simulink model "ADRCControl_CDPR_6DOF_20220708"  (R2020a)
settings: Solver=VariableStepAuto  StartTime=0.0  StopTime=12  RelTol=1e-3  EnableMultiTasking=on
values from neighbouring files (symbols this model uses):
  a = 25    [parameters_initialization.m]
  b = 0.05    [parameters_initialization.m]
  Kd = 7.062    [parameters_initialization.m]
  Kp = 70    [parameters_initialization.m]
undefined symbols (not defined in the file or in its folder): X, Y, Z
libraries: sm_lib x150, nesl_utility x52, sm_cable_robot_lib x30, simulink x1
(part 1 of 8)
settings Model: Creator=彭学东  LastModifiedBy=Administrator
settings DataIOCC: LimitDataPoints=on  MaxDataPoints=10000
settings OptimizationCC: LifeSpan=inf
settings DebuggingCC: AllowSymbolicDim=off  SFUnexpectedBacktrackingDiag=warning  SFNoUnconditionalDefaultTransitionDiag=warning  SFExecutionAtInitializationDiag=none  ArithmeticOperatorsInVariantConditions=warning
settings SFSimCC: SimUseLocalCustomCode=off  CustomCodeUndefinedFunction=UseInterfaceOnly
settings RTWCC: RTWUseLocalCustomCode=off
settings CodeAppCC: StateflowObjectComments=on
settings GRTTargetCC: TargetLangStandard=C89/C90 (ANSI)
settings ConfigComp: CovMetricSettings=dw  CovSaveCumulativeToWorkspaceVar=on  CovSaveSingleToWorkspaceVar=on  CovExternalEMLEnable=off  CovSFcnEnable=off
settings SimscapeCC: SimscapeLogType=all  SimscapeLogSimulationStatistics=on  SimscapeLogDataHistory=10000

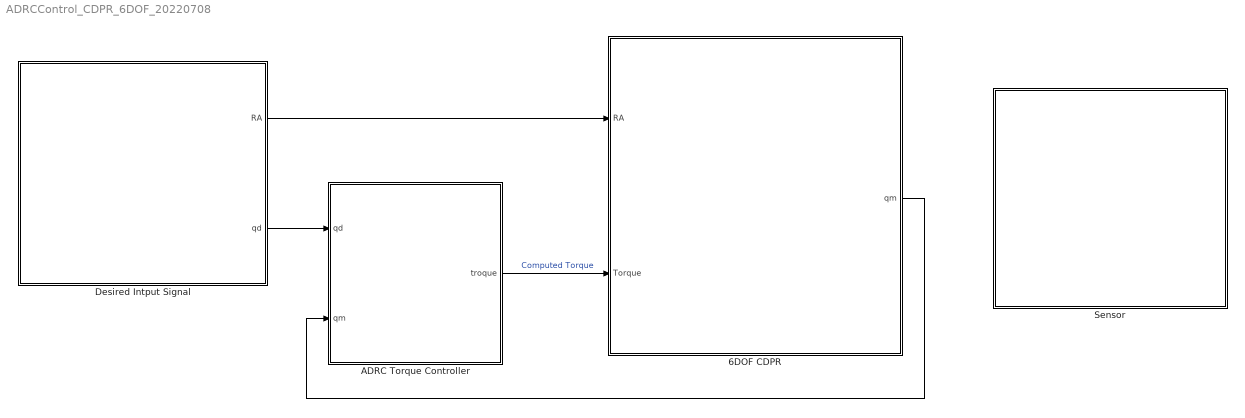
== system ADRCControl_CDPR_6DOF_20220708 ==
  6DOF CDPR : Subsystem
  ADRC Torque Controller : Subsystem
  Desired Intput Signal : Subsystem
  Sensor : Subsystem
  wires:
  Desired Intput Signal/2(qd) -> ADRC Torque Controller/1(qd)
  6DOF CDPR/1(qm) -> ADRC Torque Controller/2(qm)
  ADRC Torque Controller/1(troque) -> 6DOF CDPR/2(Torque)  "Computed Torque"
  Desired Intput Signal/1(RA) -> 6DOF CDPR/1(RA)

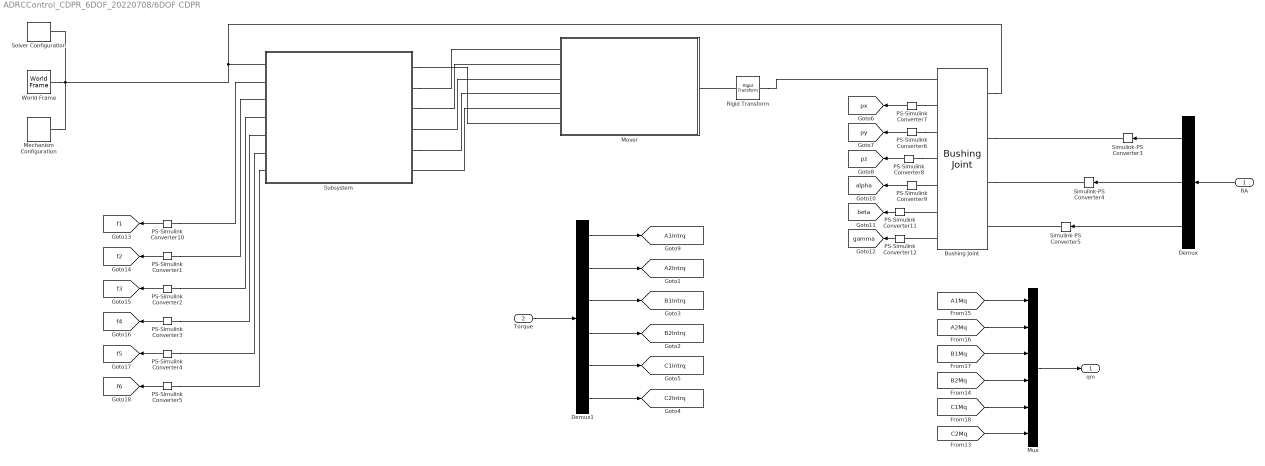
== system ADRCControl_CDPR_6DOF_20220708/6DOF CDPR ==
  RA : Inport
  Torque : Inport  Port=2
  Bushing Joint : sm_lib/Joints/Bushing Joint  JointMode=Normal  SenseConstraintForce=off  SenseConstraintForceX=off  SenseConstraintForceY=off  SenseConstraintForceZ=off  SenseConstraintTorque=off  SenseConstraintTorqueX=off  SenseConstraintTorqueY=off  SenseConstraintTorqueZ=off  SenseTotalForce=off  SenseTotalForceX=off  SenseTotalForceY=off  SenseTotalForceZ=off  SenseTotalTorque=off  SenseTotalTorqueX=off  SenseTotalTorqueY=off  SenseTotalTorqueZ=off  CompositeWrenchDir=FollowerOnBase  CompositeWrenchFrame=BaseFrame  PxEquilibriumPosition=0  PxEquilibriumPositionUnits=m  PxSpringStiffness=0  PxSpringStiffnessUnits=N/m  PxDampingCoefficient=0.1  PxDampingCoefficientUnits=N/(m/s)  PxTorqueActuationMode=NoTorque  PxMotionActuationMode=ComputedMotion  PxSensePosition=on  PxSenseVelocity=off  PxSenseAcceleration=off  PxSenseTorqueForce=off  PxSenseLowerLimitTorqueForce=off  PxSenseUpperLimitTorqueForce=off  PxLowerLimitSpecify=off  PxLowerLimitBound=-1  PxLowerLimitBoundUnits=m  PxLowerLimitStiffness=1e6  PxLowerLimitStiffnessUnits=N/m  PxLowerLimitDamping=1e3  PxLowerLimitDampingUnits=N/(m/s)  PxLowerLimitTransitionRegionWidth=1e-4  PxLowerLimitTransitionRegionWidthUnits=m  PxUpperLimitSpecify=off  PxUpperLimitBound=1  PxUpperLimitBoundUnits=m  PxUpperLimitStiffness=1e6  PxUpperLimitStiffnessUnits=N/m  PxUpperLimitDamping=1e3  PxUpperLimitDampingUnits=N/(m/s)  PxUpperLimitTransitionRegionWidth=1e-4  PxUpperLimitTransitionRegionWidthUnits=m  PxPositionTargetSpecify=on  PxPositionTargetPriority=High  PxPositionTargetValue=0.2  PxPositionTargetValueUnits=m  PxVelocityTargetSpecify=off  PxVelocityTargetPriority=High  PxVelocityTargetValue=0  PxVelocityTargetValueUnits=m/s  PyEquilibriumPosition=0  PyEquilibriumPositionUnits=m  PySpringStiffness=0  PySpringStiffnessUnits=N/m  PyDampingCoefficient=0.1  PyDampingCoefficientUnits=N/(m/s)  PyTorqueActuationMode=NoTorque  PyMotionActuationMode=ComputedMotion  PySensePosition=on  PySenseVelocity=off  PySenseAcceleration=off  PySenseTorqueForce=off  PySenseLowerLimitTorqueForce=off  PySenseUpperLimitTorqueForce=off  PyLowerLimitSpecify=off  PyLowerLimitBound=-1  PyLowerLimitBoundUnits=m  PyLowerLimitStiffness=1e6  PyLowerLimitStiffnessUnits=N/m  PyLowerLimitDamping=1e3  PyLowerLimitDampingUnits=N/(m/s)  PyLowerLimitTransitionRegionWidth=1e-4  PyLowerLimitTransitionRegionWidthUnits=m  PyUpperLimitSpecify=off  PyUpperLimitBound=1  PyUpperLimitBoundUnits=m  PyUpperLimitStiffness=1e6  PyUpperLimitStiffnessUnits=N/m  PyUpperLimitDamping=1e3  PyUpperLimitDampingUnits=N/(m/s)  PyUpperLimitTransitionRegionWidth=1e-4  PyUpperLimitTransitionRegionWidthUnits=m  PyPositionTargetSpecify=on  PyPositionTargetPriority=High  PyPositionTargetValue=0  PyPositionTargetValueUnits=m  PyVelocityTargetSpecify=off  PyVelocityTargetPriority=High  PyVelocityTargetValue=0  PyVelocityTargetValueUnits=m/s  PzEquilibriumPosition=0  PzEquilibriumPositionUnits=m  PzSpringStiffness=0  PzSpringStiffnessUnits=N/m  PzDampingCoefficient=0.1  PzDampingCoefficientUnits=N/(m/s)  PzTorqueActuationMode=NoTorque  PzMotionActuationMode=ComputedMotion  PzSensePosition=on  PzSenseVelocity=off  PzSenseAcceleration=off  PzSenseTorqueForce=off  PzSenseLowerLimitTorqueForce=off  PzSenseUpperLimitTorqueForce=off  PzLowerLimitSpecify=off  PzLowerLimitBound=-1  PzLowerLimitBoundUnits=m  PzLowerLimitStiffness=1e6  PzLowerLimitStiffnessUnits=N/m  PzLowerLimitDamping=1e3  PzLowerLimitDampingUnits=N/(m/s)  PzLowerLimitTransitionRegionWidth=1e-4  PzLowerLimitTransitionRegionWidthUnits=m  PzUpperLimitSpecify=off  PzUpperLimitBound=1  PzUpperLimitBoundUnits=m  PzUpperLimitStiffness=1e6  PzUpperLimitStiffnessUnits=N/m  PzUpperLimitDamping=1e3  PzUpperLimitDampingUnits=N/(m/s)  PzUpperLimitTransitionRegionWidth=1e-4  PzUpperLimitTransitionRegionWidthUnits=m  PzPositionTargetSpecify=on  PzPositionTargetPriority=High  PzPositionTargetValue=1.3  PzPositionTargetValueUnits=m  PzVelocityTargetSpecify=off  PzVelocityTargetPriority=High  PzVelocityTargetValue=0  PzVelocityTargetValueUnits=m/s  RxEquilibriumPosition=0  RxEquilibriumPositionUnits=deg  RxSpringStiffness=0  RxSpringStiffnessUnits=N*m/deg  RxDampingCoefficient=0.1  RxDampingCoefficientUnits=N*m/(deg/s)  RxTorqueActuationMode=ComputedTorque  RxMotionActuationMode=InputMotion  RxSensePosition=on  RxSenseVelocity=off  RxSenseAcceleration=off  RxSenseTorqueForce=off  RxSenseLowerLimitTorqueForce=off  RxSenseUpperLimitTorqueForce=off  RxLowerLimitSpecify=off  RxLowerLimitBound=-90  RxLowerLimitBoundUnits=deg  RxLowerLimitStiffness=1e4  RxLowerLimitStiffnessUnits=N*m/deg  RxLowerLimitDamping=10  RxLowerLimitDampingUnits=N*m/(deg/s)  RxLowerLimitTransitionRegionWidth=0.1  RxLowerLimitTransitionRegionWidthUnits=deg  RxUpperLimitSpecify=off  RxUpperLimitBound=90  RxUpperLimitBoundUnits=deg  RxUpperLimitStiffness=1e4  RxUpperLimitStiffnessUnits=N*m/deg  RxUpperLimitDamping=10  RxUpperLimitDampingUnits=N*m/(deg/s)  RxUpperLimitTransitionRegionWidth=0.1  RxUpperLimitTransitionRegionWidthUnits=deg  RxPositionTargetSpecify=off  RxPositionTargetPriority=High  RxPositionTargetValue=0  RxPositionTargetValueUnits=deg  RxVelocityTargetSpecify=off  RxVelocityTargetPriority=High  RxVelocityTargetValue=0  RxVelocityTargetValueUnits=deg/s  RyEquilibriumPosition=0  RyEquilibriumPositionUnits=deg  RySpringStiffness=0  RySpringStiffnessUnits=N*m/deg  RyDampingCoefficient=0.1  RyDampingCoefficientUnits=N*m/(deg/s)  RyTorqueActuationMode=ComputedTorque  RyMotionActuationMode=InputMotion  RySensePosition=on  RySenseVelocity=off  RySenseAcceleration=off  RySenseTorqueForce=off  RySenseLowerLimitTorqueForce=off  RySenseUpperLimitTorqueForce=off  RyLowerLimitSpecify=off  RyLowerLimitBound=-90  RyLowerLimitBoundUnits=deg  RyLowerLimitStiffness=1e4  RyLowerLimitStiffnessUnits=N*m/deg  RyLowerLimitDamping=10  RyLowerLimitDampingUnits=N*m/(deg/s)  RyLowerLimitTransitionRegionWidth=0.1  RyLowerLimitTransitionRegionWidthUnits=deg  RyUpperLimitSpecify=off  RyUpperLimitBound=90  RyUpperLimitBoundUnits=deg  RyUpperLimitStiffness=1e4  RyUpperLimitStiffnessUnits=N*m/deg  RyUpperLimitDamping=10  RyUpperLimitDampingUnits=N*m/(deg/s)  RyUpperLimitTransitionRegionWidth=0.1  RyUpperLimitTransitionRegionWidthUnits=deg  RyPositionTargetSpecify=off  RyPositionTargetPriority=High  RyPositionTargetValue=0  RyPositionTargetValueUnits=deg  RyVelocityTargetSpecify=off  RyVelocityTargetPriority=High  RyVelocityTargetValue=0  RyVelocityTargetValueUnits=deg/s  RzEquilibriumPosition=0  RzEquilibriumPositionUnits=deg  RzSpringStiffness=0  RzSpringStiffnessUnits=N*m/deg  RzDampingCoefficient=0.1  RzDampingCoefficientUnits=N*m/(deg/s)  RzTorqueActuationMode=ComputedTorque  RzMotionActuationMode=InputMotion  RzSensePosition=on  RzSenseVelocity=off  RzSenseAcceleration=off  RzSenseTorqueForce=off  RzSenseLowerLimitTorqueForce=off  RzSenseUpperLimitTorqueForce=off  RzLowerLimitSpecify=off  RzLowerLimitBound=-90  RzLowerLimitBoundUnits=deg  RzLowerLimitStiffness=1e4  RzLowerLimitStiffnessUnits=N*m/deg  RzLowerLimitDamping=10  RzLowerLimitDampingUnits=N*m/(deg/s)  RzLowerLimitTransitionRegionWidth=0.1  RzLowerLimitTransitionRegionWidthUnits=deg  RzUpperLimitSpecify=off  RzUpperLimitBound=90  RzUpperLimitBoundUnits=deg  RzUpperLimitStiffness=1e4  RzUpperLimitStiffnessUnits=N*m/deg  RzUpperLimitDamping=10  RzUpperLimitDampingUnits=N*m/(deg/s)  RzUpperLimitTransitionRegionWidth=0.1  RzUpperLimitTransitionRegionWidthUnits=deg  RzPositionTargetSpecify=off  RzPositionTargetPriority=High  RzPositionTargetValue=0  RzPositionTargetValueUnits=deg  RzVelocityTargetSpecify=off  RzVelocityTargetPriority=High  RzVelocityTargetValue=0  RzVelocityTargetValueUnits=deg/s
  Demux : Demux  Outputs=3
  Demux1 : Demux  Outputs=6
  Mechanism Configuration : sm_lib/Utilities/Mechanism Configuration  UniformGravity=Constant  GravityVector=[0 0 -9.80665]  GravityUnits=m/s^2  LinearizationDelta=0.001
  Mover : Subsystem
  Mux : Mux  Inputs=6
  PS-Simulink Converter{1..12} (12 alike) : nesl_utility/PS-Simulink Converter  PhysicalDomain=network_engine_domain  SubClassName=ps_output  LeftPortType=input  RightPortType=output  PseudoPeriodic=off  Frequencies=[]  Unit=inherit  AffineConversion=off
  Rigid Transform : sm_lib/Frames and Transforms/Rigid Transform  TranslationMethod=None  TranslationStandardOffset=0  TranslationLengthUnit=m  TranslationStandardAxis=+Z  TranslationCartesianOffset=[0 0 0]  TranslationROffset=0  TranslationROffsetUnits=m  TranslationZOffset=0  TranslationZOffsetUnits=m  TranslationThetaOffset=0  TranslationThetaOffsetUnits=deg  RotationMethod=ArbitraryAxis  RotationAngleUnits=deg  RotationStandardAxis=+Z  RotationAngle=120.0  RotationArbitraryAxis=[0 0 1]  FollAlignAxisA=+X  BaseAlignAxisA=+Y  FollAlignAxisB=+Y  BaseAlignAxisB=+Z  RotationSequenceAxes=FollowerAxes  RotationSequence=XYX  RotationSequenceAngles=[0 0 0]  RotationSequenceAnglesUnits=deg  RotationMatrix=[1 0 0; 0 1 0; 0 0 1]
  Simulink-PS Converter3 : nesl_utility/Simulink-PS Converter  PhysicalDomain=network_engine_domain  SubClassName=ps_input  LeftPortType=input  RightPortType=output  PseudoPeriodic=off  Frequencies=[]  NoiseDistribution=none  NoiseParameters=[]  Unit=1  AffineConversion=off  FilteringAndDerivatives=filter  SimscapeFilterOrder=2  InputFilterTimeConstant=0.001  UdotUserProvided=0
  Simulink-PS Converter4 : nesl_utility/Simulink-PS Converter  PhysicalDomain=network_engine_domain  SubClassName=ps_input  LeftPortType=input  RightPortType=output  PseudoPeriodic=off  Frequencies=[]  NoiseDistribution=none  NoiseParameters=[]  Unit=1  AffineConversion=off  FilteringAndDerivatives=filter  SimscapeFilterOrder=2  InputFilterTimeConstant=0.001  UdotUserProvided=0
  Simulink-PS Converter5 : nesl_utility/Simulink-PS Converter  PhysicalDomain=network_engine_domain  SubClassName=ps_input  LeftPortType=input  RightPortType=output  PseudoPeriodic=off  Frequencies=[]  NoiseDistribution=none  NoiseParameters=[]  Unit=1  AffineConversion=off  FilteringAndDerivatives=filter  SimscapeFilterOrder=2  InputFilterTimeConstant=0.001  UdotUserProvided=0
  Solver Configuration : nesl_utility/Solver Configuration  PhysicalDomain=network_engine_domain  SubClassName=solver  LeftPortType=input  RightPortType=generic  Tones=[]  Harmonics=[]  SimulateNoise=off  Profile=off  UseLocalSampling=off  EnableSwitchedLinearOptims=on  FrequencyDomain=off  UseCCode=off  RelTol=0.001  AbsTol=1e-06  MinStep=1e-09  ToWorkspace=off  RevertToSquareIcSolve=off  NumHomotopyIterations=100  PhasorMode=off  PhasorModeNumHarmonics=1  DoDC=off  ResidualTolerance=1e-01  UseLocalSolver=off  LocalSolverChoice=NE_BACKWARD_EULER_ADVANCER  LocalSolverSampleTime=0.001  DoFixedCost=off  MaxNonlinIter=3  MaxModeIter=2  LinearAlgebra=Sparse  EquationFormulation=NE_TIME_EF  DelaysMemoryBudget=1024  AutomaticFiltering=on  FilteringTimeConstant=0.001  PartitionStorageMethod=AS_NEEDED  PartitionMemoryBudget=1024  PartitionMethod=FAST
  Subsystem : Subsystem
  World Frame : sm_lib/Frames and Transforms/World Frame
  qm : Outport
  tag scope: A1Intrq=global, A2Intrq=global, B1Intrq=global, B2Intrq=global, C1Intrq=global, C2Intrq=global, alpha=global, beta=global, f1=global, f2=global, f3=global, f4=global, f5=global, f6=global, gamma=global, px=global, py=global, pz=global
  wires:
  PS-Simulink Converter9/1 -> [alpha]
  PS-Simulink Converter3/1 -> [f4]
  Demux1/1 -> [A1Intrq]
  Demux1/5 -> [C1Intrq]
  PS-Simulink Converter7/1 -> [px]
  PS-Simulink Converter1/1 -> [f2]
  Torque/1 -> Demux1/1
  Demux/2 -> Simulink-PS Converter4/1
  Demux/1 -> Simulink-PS Converter3/1
  PS-Simulink Converter10/1 -> [f1]
  Demux/3 -> Simulink-PS Converter5/1
  Demux1/3 -> [B1Intrq]
  PS-Simulink Converter11/1 -> [beta]
  PS-Simulink Converter8/1 -> [pz]
  Demux1/6 -> [C2Intrq]
  Demux1/2 -> [A2Intrq]
  PS-Simulink Converter2/1 -> [f3]
  PS-Simulink Converter12/1 -> [gamma]
  PS-Simulink Converter4/1 -> [f5]
  RA/1 -> Demux/1
  PS-Simulink Converter5/1 -> [f6]
  PS-Simulink Converter6/1 -> [py]
  Demux1/4 -> [B2Intrq]
  [B1Mq] -> Mux/3
  [A2Mq] -> Mux/2
  [C1Mq] -> Mux/5
  [A1Mq] -> Mux/1
  [C2Mq] -> Mux/6
  [B2Mq] -> Mux/4
  Mux/1 -> qm/1
  connections:
  World Frame/RConn1 -- Bushing Joint/LConn1 -- Subsystem/LConn1 -- Mechanism Configuration/RConn1 -- Solver Configuration/RConn1
  Subsystem/RConn2 -- Mover/LConn1
  Mover/LConn5 -- Subsystem/RConn6
  Bushing Joint/RConn6 -- PS-Simulink Converter11/LConn1
  Bushing Joint/RConn7 -- PS-Simulink Converter12/LConn1
  Rigid Transform/LConn1 -- Mover/RConn1
  PS-Simulink Converter10/LConn1 -- Subsystem/LConn2
  Bushing Joint/LConn2 -- Simulink-PS Converter3/RConn1
  Mover/LConn3 -- Subsystem/RConn4
  Subsystem/RConn5 -- Mover/LConn4
  Subsystem/RConn3 -- Mover/LConn2
  PS-Simulink Converter2/LConn1 -- Subsystem/LConn4
  PS-Simulink Converter4/LConn1 -- Subsystem/LConn6
  PS-Simulink Converter8/LConn1 -- Bushing Joint/RConn4
  PS-Simulink Converter5/LConn1 -- Subsystem/LConn7
  Bushing Joint/RConn5 -- PS-Simulink Converter9/LConn1
  PS-Simulink Converter1/LConn1 -- Subsystem/LConn3
  PS-Simulink Converter3/LConn1 -- Subsystem/LConn5
  Rigid Transform/RConn1 -- Bushing Joint/RConn1
  Subsystem/RConn1 -- Mover/LConn6
  PS-Simulink Converter7/LConn1 -- Bushing Joint/RConn2
  Bushing Joint/LConn3 -- Simulink-PS Converter4/RConn1
  PS-Simulink Converter6/LConn1 -- Bushing Joint/RConn3
  Simulink-PS Converter5/RConn1 -- Bushing Joint/LConn4

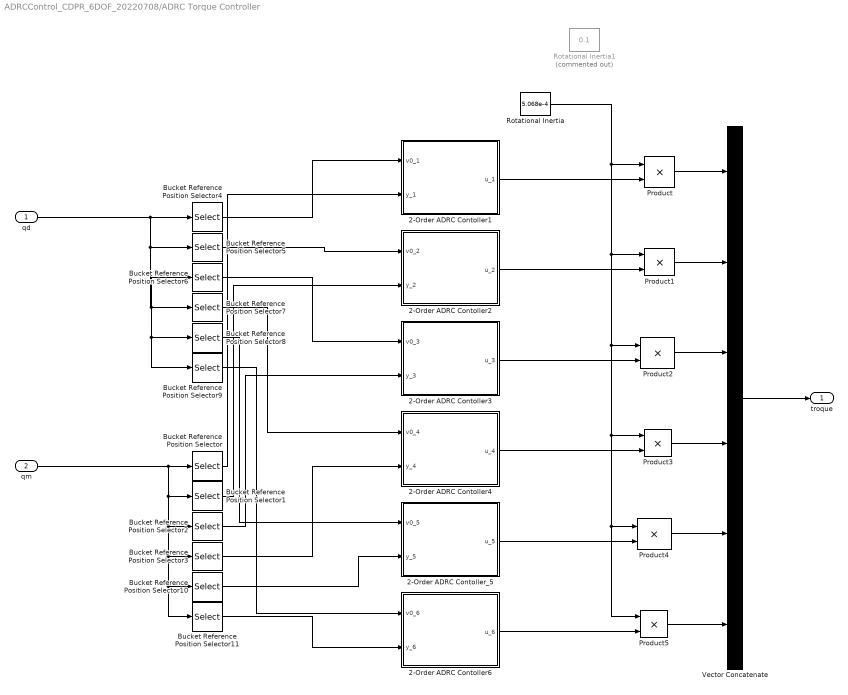
== system ADRCControl_CDPR_6DOF_20220708/ADRC Torque Controller ==
  qd : Inport
  qm : Inport  Port=2
  "2-Order ADRC Contoller1 " : Subsystem
  2-Order ADRC Contoller2 : Subsystem
  2-Order ADRC Contoller3 : Subsystem
  2-Order ADRC Contoller4 : Subsystem
  2-Order ADRC Contoller6 : Subsystem
  2-Order ADRC Contoller_5 : Subsystem
  Bucket Reference Position Selector : Selector  InputPortWidth=6  IndexOptions=Index vector (dialog)  Indices=1  OutputSizes=1
  Bucket Reference Position Selector1 : Selector  InputPortWidth=6  IndexOptions=Index vector (dialog)  Indices=2  OutputSizes=1
  Bucket Reference Position Selector10 : Selector  InputPortWidth=6  IndexOptions=Index vector (dialog)  Indices=5  OutputSizes=1
  Bucket Reference Position Selector11 : Selector  InputPortWidth=6  IndexOptions=Index vector (dialog)  Indices=6  OutputSizes=1
  Bucket Reference Position Selector2 : Selector  InputPortWidth=6  IndexOptions=Index vector (dialog)  Indices=3  OutputSizes=1
  Bucket Reference Position Selector3 : Selector  InputPortWidth=6  IndexOptions=Index vector (dialog)  Indices=4  OutputSizes=1
  Bucket Reference Position Selector4 : Selector  InputPortWidth=6  IndexOptions=Index vector (dialog)  Indices=1  OutputSizes=1
  Bucket Reference Position Selector5 : Selector  InputPortWidth=6  IndexOptions=Index vector (dialog)  Indices=2  OutputSizes=1
  Bucket Reference Position Selector6 : Selector  InputPortWidth=6  IndexOptions=Index vector (dialog)  Indices=3  OutputSizes=1
  Bucket Reference Position Selector7 : Selector  InputPortWidth=6  IndexOptions=Index vector (dialog)  Indices=4  OutputSizes=1
  Bucket Reference Position Selector8 : Selector  InputPortWidth=6  IndexOptions=Index vector (dialog)  Indices=5  OutputSizes=1
  Bucket Reference Position Selector9 : Selector  InputPortWidth=6  IndexOptions=Index vector (dialog)  Indices=6  OutputSizes=1
  Product{,1..5} (6 alike) : Product
  Rotational Inertia : Constant  Value=5.068e-4
  Rotational Inertia1 : Constant  Commented=on  Value=0.1
  Vector Concatenate : Concatenate  NumInputs=6
  troque : Outport  VectorParamsAs1DForOutWhenUnconnected=off
  wires:
  Vector Concatenate/1 -> troque/1
  Rotational Inertia/1 -> Product/1, Product1/1, Product2/1, Product3/1, Product5/1, Product4/1
  Product/1 -> Vector Concatenate/1
  Product1/1 -> Vector Concatenate/2
  Product2/1 -> Vector Concatenate/3
  Product3/1 -> Vector Concatenate/4
  "2-Order ADRC Contoller1 "/1(u_1) -> Product/2
  2-Order ADRC Contoller2/1(u_2) -> Product1/2
  2-Order ADRC Contoller3/1(u_3) -> Product2/2
  2-Order ADRC Contoller4/1(u_4) -> Product3/2
  qm/1 -> Bucket Reference Position Selector11/1, Bucket Reference Position Selector10/1, Bucket Reference Position Selector3/1, Bucket Reference Position Selector2/1, Bucket Reference Position Selector1/1, Bucket Reference Position Selector/1
  qd/1 -> Bucket Reference Position Selector9/1, Bucket Reference Position Selector8/1, Bucket Reference Position Selector7/1, Bucket Reference Position Selector6/1, Bucket Reference Position Selector5/1, Bucket Reference Position Selector4/1
  Bucket Reference Position Selector4/1 -> "2-Order ADRC Contoller1 "/1(v0_1)
  Bucket Reference Position Selector5/1 -> 2-Order ADRC Contoller2/1(v0_2)
  Bucket Reference Position Selector6/1 -> 2-Order ADRC Contoller3/1(v0_3)
  Bucket Reference Position Selector7/1 -> 2-Order ADRC Contoller4/1(v0_4)
  Bucket Reference Position Selector/1 -> "2-Order ADRC Contoller1 "/2(y_1)
  Bucket Reference Position Selector1/1 -> 2-Order ADRC Contoller2/2(y_2)
  Bucket Reference Position Selector2/1 -> 2-Order ADRC Contoller3/2(y_3)
  Bucket Reference Position Selector3/1 -> 2-Order ADRC Contoller4/2(y_4)
  Bucket Reference Position Selector8/1 -> 2-Order ADRC Contoller_5/1(v0_5)
  Bucket Reference Position Selector9/1 -> 2-Order ADRC Contoller6/1(v0_6)
  Bucket Reference Position Selector10/1 -> 2-Order ADRC Contoller_5/2(y_5)
  Bucket Reference Position Selector11/1 -> 2-Order ADRC Contoller6/2(y_6)
  Product5/1 -> Vector Concatenate/6
  2-Order ADRC Contoller_5/1(u_5) -> Product4/2
  2-Order ADRC Contoller6/1(u_6) -> Product5/2
  Product4/1 -> Vector Concatenate/5

== system ADRCControl_CDPR_6DOF_20220708/Desired Intput Signal ==
  Clock1 : Clock  Commented=on
      settings: Decimation=12
  Clock2 : Clock
      settings: Decimation=12
  Desried Angle : MATLAB Function  TreatAsAtomicUnit=on
  Desried Torque1 : MATLAB Function  Commented=on  TreatAsAtomicUnit=on
  Mux : Mux  Inputs=3
  Mux1 : Mux  Inputs=6
  Mux2 : Mux  Commented=on  Inputs=6
  Rotation Angle : Subsystem
  RA : Outport
  qd : Outport  Port=2
  wires:
  Rotation Angle/1(Out1) -> Mux/1
  Rotation Angle/2(Out2) -> Mux/2
  Rotation Angle/3(Out3) -> Mux/3
  Mux/1 -> RA/1
  Desried Angle/2(A2q) -> Mux1/2
  Desried Angle/6(C2q) -> Mux1/6
  Desried Angle/3(B1q) -> Mux1/3
  Clock2/1 -> Desried Angle/1(t)
  Desried Angle/1(A1q) -> Mux1/1
  Desried Angle/4(B2q) -> Mux1/4
  Desried Angle/5(C1q) -> Mux1/5
  Mux1/1 -> qd/1
  Desried Torque1/4(B2q) -> Mux2/4
  Desried Torque1/3(B1q) -> Mux2/3
  Desried Torque1/2(A2q) -> Mux2/2
  Desried Torque1/1(A1q) -> Mux2/1
  Desried Torque1/6(C2q) -> Mux2/6
  Desried Torque1/5(C1q) -> Mux2/5
  Clock1/1 -> Desried Torque1/1(t)

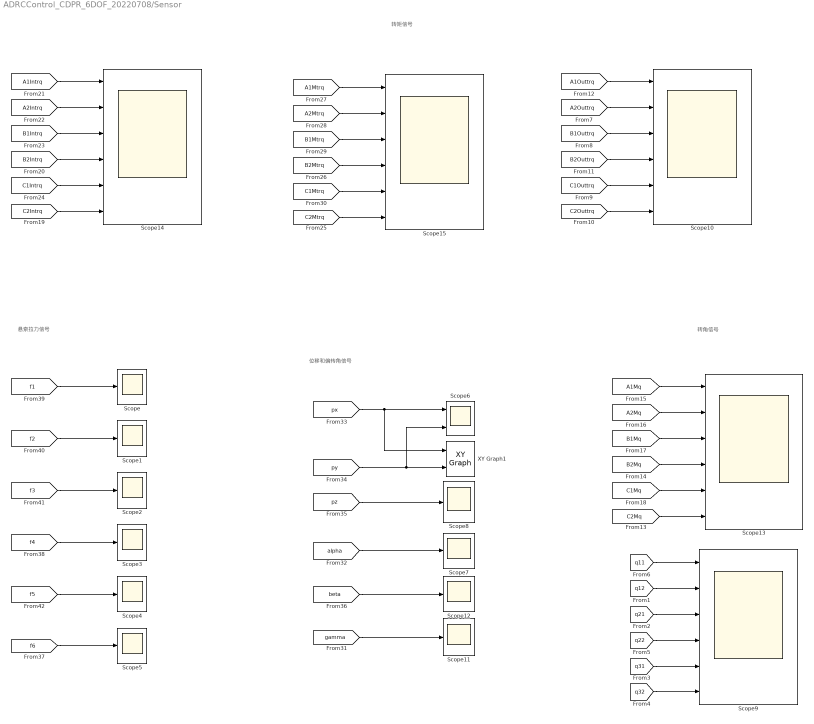
== system ADRCControl_CDPR_6DOF_20220708/Sensor ==
  note: 悬索拉力信号
  note: 位移和偏转角信号
  note: 转角信号
  note: 转矩信号
  Scope{,1..5,7..8,11..12} (10 alike) : Scope
  Scope{9..10,13..15} (5 alike) : Scope  NumInputPorts=6
  Scope6 : Scope  NumInputPorts=2
  XY Graph1 : simulink/Sinks/XY Graph  xmin=-1.1  xmax=1.1  ymin=-1.5  ymax=1.5  st=-1
  wires:
  [C2Outtrq] -> Scope10/6
  [C2Mtrq] -> Scope15/6
  [C1Intrq] -> Scope14/5
  [B2Intrq] -> Scope14/4
  [B1Mtrq] -> Scope15/3
  [C1Mtrq] -> Scope15/5
  [B1Intrq] -> Scope14/3
  [B2Mtrq] -> Scope15/4
  [A2Intrq] -> Scope14/2
  [A1Mtrq] -> Scope15/1
  [C1Outtrq] -> Scope10/5
  [A1Intrq] -> Scope14/1
  [C2Intrq] -> Scope14/6
  [B1Outtrq] -> Scope10/3
  [A2Outtrq] -> Scope10/2
  [A1Outtrq] -> Scope10/1
  [B2Outtrq] -> Scope10/4
  [A2Mtrq] -> Scope15/2
  [B1Mq] -> Scope13/3
  [B2Mq] -> Scope13/4
  [C2Mq] -> Scope13/6
  [q12] -> Scope9/2
  [q21] -> Scope9/3
  [C1Mq] -> Scope13/5
  [A1Mq] -> Scope13/1
  [q22] -> Scope9/4
  [q32] -> Scope9/6
  [q31] -> Scope9/5
  [q11] -> Scope9/1
  [A2Mq] -> Scope13/2
  [gamma] -> Scope11/1
  [beta] -> Scope12/1
  [alpha] -> Scope7/1
  [pz] -> Scope8/1
  [py] -> XY Graph1/2, Scope6/2
  [px] -> Scope6/1, XY Graph1/1
  [f1] -> Scope/1
  [f2] -> Scope1/1
  [f3] -> Scope2/1
  [f4] -> Scope3/1
  [f5] -> Scope4/1
  [f6] -> Scope5/1

== system ADRCControl_CDPR_6DOF_20220708/6DOF CDPR/Mover ==
  Extruded Solid : sm_lib/Body Elements/Extruded Solid  GraphicAmbientColor=[0.15 0.15 0.15 1.0]  BasedOnType=Mass  CenterOfMass=[0 0 0]  CenterOfMassUnits=m  GraphicDiffuseColor=[0.0 0.2 1.0]  ExportConvexHullGeometry=off  ExtrusionCrossSection=[1 1; -1 1; -1 -1; 1 -1]  ExtrusionCrossSectionUnits=m  Density=1000  DensityUnits=kg/m^3  DoExposeReferenceFrame=on  GraphicEmissiveColor=[0.0 0.0 0.0 1.0]  ExportEntireGeometry=off  ExtrusionLength=0.1  ExtrusionLengthUnits=m  ExtrusionType=Regular  SerializedFrames=<Frames><Frame><Id>Frame1</Id><Value><Name>F1</Name><Origin><Source>GeometricFeature</Source><FeatureName>side curve 3</FeatureName></Origin><PrimaryAxis><DefinedDirection>+Z</DefinedDirection><Source>ReferenceFrame</Source><SourceDirection>+Z</SourceDirection><FeatureName></FeatureName></PrimaryAxis><SecondaryAxis><DefinedDirection>+X</DefinedDirection><Source>ReferenceFrame</Source><SourceDirection>+X</SourceDirection><FeatureName></FeatureName></SecondaryAxis></Value></Frame><Frame><Id>Frame2</Id><Value><Name>F2</Name><Origin><Source>GeometricFeature</Source><FeatureName>side curve 1</FeatureName></Origin><PrimaryAxis><DefinedDirection>+Z</DefinedDirection><Source>ReferenceFrame</Source><SourceDirection>+Z</SourceDirection><FeatureName></FeatureName></PrimaryAxis><SecondaryAxis><DefinedDirection>+X</DefinedDirection><Source>ReferenceFrame</Source><SourceDirection>+X</SourceDirection><FeatureName></FeatureName></SecondaryAxis></Value></Frame><Frame><Id>Frame3</Id><Value><Name>F3</Name><Origin><Source>GeometricFeature</Source><FeatureName>side curve 2</FeatureName></Origin><PrimaryAxis><DefinedDirection>+Z</DefinedDirection><Source>ReferenceFrame</Source><SourceDirection>+Z</SourceDirection><FeatureName></FeatureName></PrimaryAxis><SecondaryAxis><DefinedDirection>+X</DefinedDirection><Source>ReferenceFrame</Source><SourceDirection>+X</SourceDirection><FeatureName></FeatureName></SecondaryAxis></Value></Frame></Frames>  MarkerShape=Sphere  MarkerSize=10  GraphicType=FromGeometry  InertiaType=Custom  Mass=5  MassUnits=kg  MomentsOfInertia=[0.001 0.001 0.03125]  MomentsOfInertiaUnits=kg*m^2  PolygonNumSides=3  GraphicOpacity=1.0  PolygonOuterRadius=0.088  PolygonOuterRadiusUnits=m  ProductsOfInertia=[0 0 0]  ProductsOfInertiaUnits=kg*m^2  GraphicShininess=75  GraphicSpecularColor=[0.5 0.5 0.5 1.0]  GraphicVisPropType=SimpleVisualProperties
  1 : PMIOPort  Side=Left
  2 : PMIOPort  Port=2  Side=Left
  3 : PMIOPort  Port=3  Side=Left
  4 : PMIOPort  Port=4  Side=Left
  5 : PMIOPort  Port=5  Side=Left
  6 : PMIOPort  Port=6  Side=Left
  B : PMIOPort  Port=7  Side=Right
  connections:
  5/RConn1 -- 6/RConn1 -- Extruded Solid/RConn2
  3/RConn1 -- 4/RConn1 -- Extruded Solid/LConn2
  2/RConn1 -- 1/RConn1 -- Extruded Solid/LConn1
  B/RConn1 -- Extruded Solid/RConn1

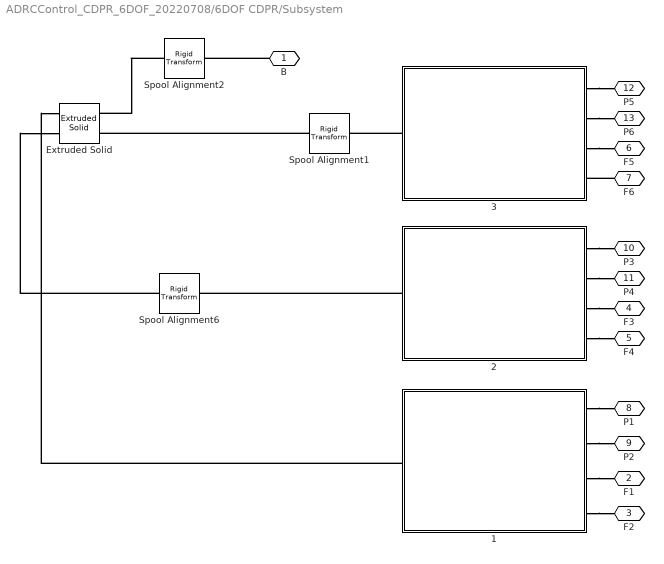
== system ADRCControl_CDPR_6DOF_20220708/6DOF CDPR/Subsystem ==
  1 : Subsystem
  2 : Subsystem
  3 : Subsystem
  Extruded Solid : sm_lib/Body Elements/Extruded Solid  GraphicAmbientColor=[0.15 0.15 0.15 1.0]  BasedOnType=Density  CenterOfMass=[0 0 0]  CenterOfMassUnits=m  GraphicDiffuseColor=[0.5 0.5 0.5]  ExportConvexHullGeometry=off  ExtrusionCrossSection=[1 1; -1 1; -1 -1; 1 -1]  ExtrusionCrossSectionUnits=m  Density=1000  DensityUnits=kg/m^3  DoExposeReferenceFrame=on  GraphicEmissiveColor=[0.0 0.0 0.0 1.0]  ExportEntireGeometry=off  ExtrusionLength=0.2  ExtrusionLengthUnits=m  ExtrusionType=Regular  SerializedFrames=<Frames><Frame><Id>Frame1</Id><Value><Name>F1</Name><Origin><Source>GeometricFeature</Source><FeatureName>top point 3</FeatureName></Origin><PrimaryAxis><DefinedDirection>+Z</DefinedDirection><Source>ReferenceFrame</Source><SourceDirection>+Z</SourceDirection><FeatureName></FeatureName></PrimaryAxis><SecondaryAxis><DefinedDirection>+X</DefinedDirection><Source>ReferenceFrame</Source><SourceDirection>+X</SourceDirection><FeatureName></FeatureName></SecondaryAxis></Value></Frame><Frame><Id>Frame2</Id><Value><Name>F2</Name><Origin><Source>GeometricFeature</Source><FeatureName>top point 1</FeatureName></Origin><PrimaryAxis><DefinedDirection>+Z</DefinedDirection><Source>ReferenceFrame</Source><SourceDirection>+Z</SourceDirection><FeatureName></FeatureName></PrimaryAxis><SecondaryAxis><DefinedDirection>+X</DefinedDirection><Source>ReferenceFrame</Source><SourceDirection>+X</SourceDirection><FeatureName></FeatureName></SecondaryAxis></Value></Frame><Frame><Id>Frame3</Id><Value><Name>F3</Name><Origin><Source>GeometricFeature</Source><FeatureName>top point 2</FeatureName></Origin><PrimaryAxis><DefinedDirection>+Z</DefinedDirection><Source>ReferenceFrame</Source><SourceDirection>+Z</SourceDirection><FeatureName></FeatureName></PrimaryAxis><SecondaryAxis><DefinedDirection>+X</DefinedDirection><Source>ReferenceFrame</Source><SourceDirection>+X</SourceDirection><FeatureName></FeatureName></SecondaryAxis></Value></Frame></Frames>  MarkerShape=Sphere  MarkerSize=10  GraphicType=FromGeometry  InertiaType=CalculateFromGeometry  Mass=1  MassUnits=kg  MomentsOfInertia=[1 1 1]  MomentsOfInertiaUnits=kg*m^2  PolygonNumSides=3  GraphicOpacity=1.0  PolygonOuterRadius=2.254  PolygonOuterRadiusUnits=m  ProductsOfInertia=[0 0 0]  ProductsOfInertiaUnits=kg*m^2  GraphicShininess=75  GraphicSpecularColor=[0.5 0.5 0.5 1.0]  GraphicVisPropType=SimpleVisualProperties
  Spool Alignment1 : sm_lib/Frames and Transforms/Rigid Transform  TranslationMethod=None  TranslationStandardOffset=0  TranslationLengthUnit=m  TranslationStandardAxis=+Z  TranslationCartesianOffset=[0 0 0]  TranslationROffset=0  TranslationROffsetUnits=m  TranslationZOffset=0  TranslationZOffsetUnits=m  TranslationThetaOffset=0  TranslationThetaOffsetUnits=deg  RotationMethod=ArbitraryAxis  RotationAngleUnits=deg  RotationStandardAxis=+Z  RotationAngle=-120.0  RotationArbitraryAxis=[0 0 1]  FollAlignAxisA=+X  BaseAlignAxisA=+X  FollAlignAxisB=+Y  BaseAlignAxisB=+Y  RotationSequenceAxes=FollowerAxes  RotationSequence=XYX  RotationSequenceAngles=[0 0 0]  RotationSequenceAnglesUnits=deg  RotationMatrix=[1 0 0; 0 1 0; 0 0 1]
  Spool Alignment2 : sm_lib/Frames and Transforms/Rigid Transform  TranslationMethod=None  TranslationStandardOffset=0  TranslationLengthUnit=m  TranslationStandardAxis=+Z  TranslationCartesianOffset=[0 0 0]  TranslationROffset=0  TranslationROffsetUnits=m  TranslationZOffset=0  TranslationZOffsetUnits=m  TranslationThetaOffset=0  TranslationThetaOffsetUnits=deg  RotationMethod=ArbitraryAxis  RotationAngleUnits=deg  RotationStandardAxis=+Z  RotationAngle=180.0  RotationArbitraryAxis=[0 0 1]  FollAlignAxisA=+X  BaseAlignAxisA=+X  FollAlignAxisB=+Y  BaseAlignAxisB=+Y  RotationSequenceAxes=FollowerAxes  RotationSequence=XYX  RotationSequenceAngles=[0 0 0]  RotationSequenceAnglesUnits=deg  RotationMatrix=[1 0 0; 0 1 0; 0 0 1]
  Spool Alignment6 : sm_lib/Frames and Transforms/Rigid Transform  TranslationMethod=None  TranslationStandardOffset=0  TranslationLengthUnit=m  TranslationStandardAxis=+Z  TranslationCartesianOffset=[0 0 0]  TranslationROffset=0  TranslationROffsetUnits=m  TranslationZOffset=0  TranslationZOffsetUnits=m  TranslationThetaOffset=0  TranslationThetaOffsetUnits=deg  RotationMethod=ArbitraryAxis  RotationAngleUnits=deg  RotationStandardAxis=+Z  RotationAngle=120.0  RotationArbitraryAxis=[0 0 1]  FollAlignAxisA=+X  BaseAlignAxisA=+X  FollAlignAxisB=+Y  BaseAlignAxisB=+Y  RotationSequenceAxes=FollowerAxes  RotationSequence=XYX  RotationSequenceAngles=[0 0 0]  RotationSequenceAnglesUnits=deg  RotationMatrix=[1 0 0; 0 1 0; 0 0 1]
  B : PMIOPort  Side=Left
  F1 : PMIOPort  Port=2  Side=Left
  F2 : PMIOPort  Port=3  Side=Left
  F3 : PMIOPort  Port=4  Side=Left
  F4 : PMIOPort  Port=5  Side=Left
  F5 : PMIOPort  Port=6  Side=Left
  F6 : PMIOPort  Port=7  Side=Left
  P1 : PMIOPort  Port=8  Side=Right
  P2 : PMIOPort  Port=9  Side=Right
  P3 : PMIOPort  Port=10  Side=Right
  P4 : PMIOPort  Port=11  Side=Right
  P5 : PMIOPort  Port=12  Side=Right
  P6 : PMIOPort  Port=13  Side=Right
  connections:
  1/LConn1 -- Extruded Solid/LConn1
  1/RConn1 -- P1/RConn1
  3/RConn1 -- P5/RConn1
  3/LConn1 -- Spool Alignment1/RConn1
  Spool Alignment6/LConn1 -- Extruded Solid/LConn2
  Spool Alignment1/LConn1 -- Extruded Solid/RConn2
  2/LConn1 -- Spool Alignment6/RConn1
  2/RConn1 -- P3/RConn1
  3/RConn2 -- P6/RConn1
  2/RConn2 -- P4/RConn1
  1/RConn2 -- P2/RConn1
  3/RConn3 -- F5/RConn1
  F6/RConn1 -- 3/RConn4
  2/RConn3 -- F3/RConn1
  2/RConn4 -- F4/RConn1
  1/RConn4 -- F2/RConn1
  1/RConn3 -- F1/RConn1
  B/RConn1 -- Spool Alignment2/RConn1
  Spool Alignment2/LConn1 -- Extruded Solid/RConn1

== system ADRCControl_CDPR_6DOF_20220708/ADRC Torque Controller/2-Order ADRC Contoller1  ==
  v0_1 : Inport
  y_1 : Inport  Port=2
  1/b0 : Gain  Gain=1/b
  3-order ESO : Subsystem
  Constant3 : Constant  Value=a
  ESO parameters assignment : MATLAB Function  TreatAsAtomicUnit=on
  PD : Subsystem
  Sum : Sum  Inputs=|+-
  Sum1 : Sum  Inputs=|+-
  b0 : Gain  Gain=b
  u_1 : Outport  VectorParamsAs1DForOutWhenUnconnected=off
  wires:
  1/b0/1 -> u_1/1, b0/1
  ESO parameters assignment/1(beta01) -> 3-order ESO/3(beta01)
  Sum1/1 -> 1/b0/1
  ESO parameters assignment/3(beta03) -> 3-order ESO/5(beta03)
  ESO parameters assignment/2(beta02) -> 3-order ESO/4(beta02)
  b0/1 -> 3-order ESO/2(u)
  Constant3/1 -> ESO parameters assignment/1(omega)
  y_1/1 -> 3-order ESO/1(y)
  3-order ESO/1(z1) -> Sum/2
  v0_1/1 -> Sum/1
  Sum/1 -> PD/1(e)
  3-order ESO/2(z2) -> PD/2(Z2)
  PD/1(u0) -> Sum1/1
  3-order ESO/3(z3) -> Sum1/2

== system ADRCControl_CDPR_6DOF_20220708/ADRC Torque Controller/2-Order ADRC Contoller2 ==
  v0_2 : Inport
  y_2 : Inport  Port=2
  1/b0 : Gain  Gain=1/b
  3-order ESO : Subsystem
  Constant3 : Constant  Value=a
  ESO parameters assignment : MATLAB Function  TreatAsAtomicUnit=on
  PD : Subsystem
  Sum : Sum  Inputs=|+-
  Sum1 : Sum  Inputs=|+-
  b0 : Gain  Gain=b
  u_2 : Outport  VectorParamsAs1DForOutWhenUnconnected=off
  wires:
  1/b0/1 -> u_2/1, b0/1
  ESO parameters assignment/1(beta01) -> 3-order ESO/3(beta01)
  Sum1/1 -> 1/b0/1
  ESO parameters assignment/3(beta03) -> 3-order ESO/5(beta03)
  ESO parameters assignment/2(beta02) -> 3-order ESO/4(beta02)
  b0/1 -> 3-order ESO/2(u)
  Constant3/1 -> ESO parameters assignment/1(omega)
  y_2/1 -> 3-order ESO/1(y)
  3-order ESO/1(z1) -> Sum/2
  v0_2/1 -> Sum/1
  Sum/1 -> PD/1(e)
  3-order ESO/2(z2) -> PD/2(Z2)
  PD/1(u0) -> Sum1/1
  3-order ESO/3(z3) -> Sum1/2

== system ADRCControl_CDPR_6DOF_20220708/ADRC Torque Controller/2-Order ADRC Contoller3 ==
  v0_3 : Inport
  y_3 : Inport  Port=2
  1/b0 : Gain  Gain=1/b
  3-order ESO : Subsystem
  Constant3 : Constant  Value=a
  ESO parameters assignment : MATLAB Function  TreatAsAtomicUnit=on
  PD : Subsystem
  Sum : Sum  Inputs=|+-
  Sum1 : Sum  Inputs=|+-
  b0 : Gain  Gain=b
  u_3 : Outport  VectorParamsAs1DForOutWhenUnconnected=off
  wires:
  1/b0/1 -> u_3/1, b0/1
  ESO parameters assignment/1(beta01) -> 3-order ESO/3(beta01)
  Sum1/1 -> 1/b0/1
  ESO parameters assignment/3(beta03) -> 3-order ESO/5(beta03)
  ESO parameters assignment/2(beta02) -> 3-order ESO/4(beta02)
  b0/1 -> 3-order ESO/2(u)
  Constant3/1 -> ESO parameters assignment/1(omega)
  y_3/1 -> 3-order ESO/1(y)
  3-order ESO/1(z1) -> Sum/2
  v0_3/1 -> Sum/1
  Sum/1 -> PD/1(e)
  3-order ESO/2(z2) -> PD/2(Z2)
  PD/1(u0) -> Sum1/1
  3-order ESO/3(z3) -> Sum1/2

== system ADRCControl_CDPR_6DOF_20220708/ADRC Torque Controller/2-Order ADRC Contoller4 ==
  v0_4 : Inport
  y_4 : Inport  Port=2
  1/b0 : Gain  Gain=1/b
  3-order ESO : Subsystem
  Constant3 : Constant  Value=a
  ESO parameters assignment : MATLAB Function  TreatAsAtomicUnit=on
  PD : Subsystem
  Sum : Sum  Inputs=|+-
  Sum1 : Sum  Inputs=|+-
  b0 : Gain  Gain=b
  u_4 : Outport  VectorParamsAs1DForOutWhenUnconnected=off
  wires:
  1/b0/1 -> u_4/1, b0/1
  ESO parameters assignment/1(beta01) -> 3-order ESO/3(beta01)
  Sum1/1 -> 1/b0/1
  ESO parameters assignment/3(beta03) -> 3-order ESO/5(beta03)
  ESO parameters assignment/2(beta02) -> 3-order ESO/4(beta02)
  b0/1 -> 3-order ESO/2(u)
  Constant3/1 -> ESO parameters assignment/1(omega)
  y_4/1 -> 3-order ESO/1(y)
  3-order ESO/1(z1) -> Sum/2
  v0_4/1 -> Sum/1
  Sum/1 -> PD/1(e)
  3-order ESO/2(z2) -> PD/2(Z2)
  PD/1(u0) -> Sum1/1
  3-order ESO/3(z3) -> Sum1/2

== system ADRCControl_CDPR_6DOF_20220708/ADRC Torque Controller/2-Order ADRC Contoller6 ==
  v0_6 : Inport
  y_6 : Inport  Port=2
  1/b0 : Gain  Gain=1/b
  3-order ESO : Subsystem
  Constant3 : Constant  Value=a
  ESO parameters assignment : MATLAB Function  TreatAsAtomicUnit=on
  PD : Subsystem
  Sum : Sum  Inputs=|+-
  Sum1 : Sum  Inputs=|+-
  b0 : Gain  Gain=b
  u_6 : Outport  VectorParamsAs1DForOutWhenUnconnected=off
  wires:
  1/b0/1 -> u_6/1, b0/1
  ESO parameters assignment/1(beta01) -> 3-order ESO/3(beta01)
  Sum1/1 -> 1/b0/1
  ESO parameters assignment/3(beta03) -> 3-order ESO/5(beta03)
  ESO parameters assignment/2(beta02) -> 3-order ESO/4(beta02)
  b0/1 -> 3-order ESO/2(u)
  Constant3/1 -> ESO parameters assignment/1(omega)
  y_6/1 -> 3-order ESO/1(y)
  3-order ESO/1(z1) -> Sum/2
  v0_6/1 -> Sum/1
  Sum/1 -> PD/1(e)
  3-order ESO/2(z2) -> PD/2(Z2)
  PD/1(u0) -> Sum1/1
  3-order ESO/3(z3) -> Sum1/2

== system ADRCControl_CDPR_6DOF_20220708/ADRC Torque Controller/2-Order ADRC Contoller_5 ==
  v0_5 : Inport
  y_5 : Inport  Port=2
  1/b0 : Gain  Gain=1/b
  3-order ESO : Subsystem
  Constant3 : Constant  Value=a
  ESO parameters assignment : MATLAB Function  TreatAsAtomicUnit=on
  PD : Subsystem
  Sum : Sum  Inputs=|+-
  Sum1 : Sum  Inputs=|+-
  b0 : Gain  Gain=b
  u_5 : Outport  VectorParamsAs1DForOutWhenUnconnected=off
  wires:
  1/b0/1 -> u_5/1, b0/1
  ESO parameters assignment/1(beta01) -> 3-order ESO/3(beta01)
  Sum1/1 -> 1/b0/1
  ESO parameters assignment/3(beta03) -> 3-order ESO/5(beta03)
  ESO parameters assignment/2(beta02) -> 3-order ESO/4(beta02)
  b0/1 -> 3-order ESO/2(u)
  Constant3/1 -> ESO parameters assignment/1(omega)
  y_5/1 -> 3-order ESO/1(y)
  3-order ESO/1(z1) -> Sum/2
  v0_5/1 -> Sum/1
  Sum/1 -> PD/1(e)
  3-order ESO/2(z2) -> PD/2(Z2)
  PD/1(u0) -> Sum1/1
  3-order ESO/3(z3) -> Sum1/2

== system ADRCControl_CDPR_6DOF_20220708/Desired Intput Signal/Rotation Angle ==
  Constant3 : Constant  Value=0
  Constant4 : Constant  Value=0
  Constant5 : Constant  Value=0
  Sum3 : Sum  Inputs=|+-
  Sum4 : Sum  Inputs=|+-
  Sum5 : Sum  Inputs=|+-
  Out1 : Outport
  Out2 : Outport  Port=2
  Out3 : Outport  Port=3
  wires:
  Constant3/1 -> Sum3/1
  Constant4/1 -> Sum4/1
  Sum4/1 -> Out2/1
  Constant5/1 -> Sum5/1
  Sum3/1 -> Out1/1
  Sum5/1 -> Out3/1
  [gamma] -> Sum5/2
  [beta] -> Sum4/2
  [alpha] -> Sum3/2
